simulink model "BBBC_5"  (R2022b)
settings: Solver=VariableStepAuto  StartTime=0.0  StopTime=5  RelTol=1e-3
undefined symbols (not defined in the file): dct, dEv, Ev, sigbuilder_block
libraries: simulink x6, spsMosfetLib x4, spsSeriesRLCBranchLib x4, spsCurrentMeasurementLib x2, spsVoltageMeasurementLib x2, spsGroundLib x1, spsControlledVoltageSourceLib x1, spspowerguiLib x1
settings Model: Creator=Dopechuro  LastModifiedBy=Dopechuro

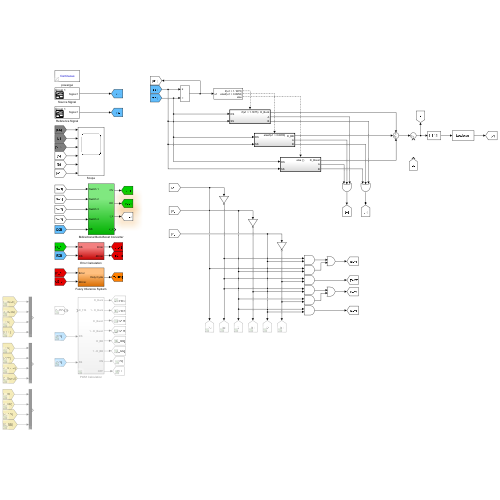
[thumbnail: Simulink's stored preview of the top-level diagram]
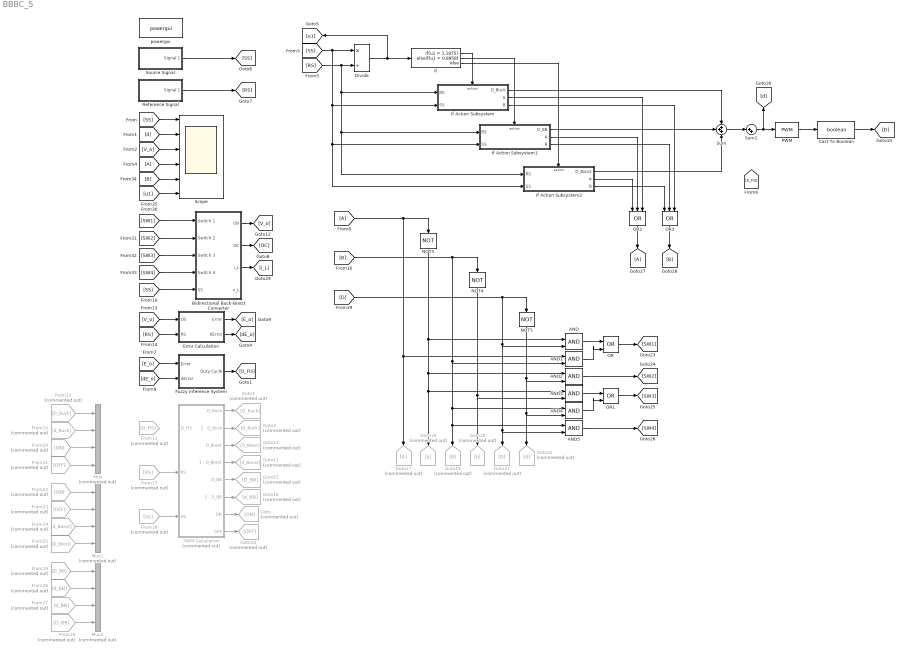
== system BBBC_5 ==
  AND{,1..5} (6 alike) : Logic  IconShape=distinctive  AllPortsSameDT=off  OutDataTypeStr=boolean
  Bidirectional Buck-Boost Converter : Subsystem
  Cast To Boolean : DataTypeConversion  OutDataTypeStr=boolean  SaturateOnIntegerOverflow=off  RndMeth=Floor
  Divide : Product  Inputs=*/
  Error Calculation : Subsystem
  From11 : From  Commented=on  GotoTag=D_FIS
  From12 : From  Commented=on  GotoTag=D_Buck
  From15 : From  Commented=on  GotoTag=d_Buck
  From17 : From  Commented=on  GotoTag=RS
  From18 : From  Commented=on  GotoTag=SS
  From19 : From  Commented=on  GotoTag=D_BB
  From20 : From  Commented=on  GotoTag=ON
  From21 : From  Commented=on  GotoTag=OFF
  From22 : From  Commented=on  GotoTag=ON
  From23 : From  Commented=on  GotoTag=OFF
  From24 : From  Commented=on  GotoTag=d_Boost
  From25 : From  Commented=on  GotoTag=D_Boost
  From26 : From  Commented=on  GotoTag=d_BB
  From27 : From  Commented=on  GotoTag=d_BB
  From28 : From  Commented=on  GotoTag=D_BB
  From4 : From
  From8 : From
  Fuzzy Inference System : Subsystem
  Goto : Goto  Commented=on  GotoTag=ON
  Goto11 : Goto  Commented=on  GotoTag=d_Boost
  Goto13 : Goto  Commented=on  GotoTag=D_Boost
  Goto14 : Goto  Commented=on  GotoTag=OFF
  Goto15 : Goto  Commented=on  GotoTag=D_BB
  Goto16 : Goto  Commented=on  GotoTag=d_BB
  Goto17 : Goto  Commented=on
  Goto18 : Goto  Commented=on  GotoTag=a
  Goto19 : Goto  Commented=on  GotoTag=B
  Goto2 : Goto  Commented=on  GotoTag=d_Buck
  Goto20 : Goto  Commented=on  GotoTag=b
  Goto21 : Goto  Commented=on  GotoTag=D
  Goto22 : Goto  Commented=on  GotoTag=d
  Goto27 : Goto
  Goto3 : Goto  Commented=on  GotoTag=D_Buck
  If : If  IfExpression=u1 > 1.1875  ElseIfExpressions=u1 > 0.8958
  If Action Subsystem : Subsystem  TreatAsAtomicUnit=on
  If Action Subsystem1 : Subsystem  TreatAsAtomicUnit=on
  If Action Subsystem2 : Subsystem  TreatAsAtomicUnit=on
  Mux : Mux  Commented=on
  Mux1 : Mux  Commented=on
  Mux2 : Mux  Commented=on
  NOT3 : Logic  Operator=NOT  IconShape=distinctive  AllPortsSameDT=off  OutDataTypeStr=boolean
  NOT4 : Logic  Operator=NOT  IconShape=distinctive  AllPortsSameDT=off  OutDataTypeStr=boolean
  NOT5 : Logic  Operator=NOT  IconShape=distinctive  AllPortsSameDT=off  OutDataTypeStr=boolean
  OR : Logic  Operator=OR  IconShape=distinctive  AllPortsSameDT=off  OutDataTypeStr=boolean
  OR1 : Logic  Operator=OR  IconShape=distinctive  AllPortsSameDT=off  OutDataTypeStr=boolean
  OR2 : Logic  Operator=OR  Inputs=3  IconShape=distinctive  AllPortsSameDT=off  OutDataTypeStr=boolean
  OR3 : Logic  Operator=OR  Inputs=3  IconShape=distinctive  AllPortsSameDT=off  OutDataTypeStr=boolean
  PWM : simulink/Discontinuities/PWM  DisableCoverage=on  Period=1e-5  InitialDelay=0  DisallowZeroDutyCycle=off  RunAtFixedTimeIntervals=off  SampleTime=0.1
  PWM Calculation : Subsystem  Commented=on
  Reference Signal : Subsystem  Tag=STV Subsys  LoadFcn=sigbuilder_block('load');  StartFcn=sigbuilder_block('start');  StopFcn=sigbuilder_block('stop');  ClipboardFcn=sigbuilder_block('clipboard');  mask(Sigbuilder block){tuvar=[0:10]}
      mask help: Simulink:masks:SigbuilderBlock_MD
      mask init:
      | if ~strcmp(get_param(bdroot(gcbh),'SimulationStatus'),'stopped') tuvar = sigbuilder_block('maskInit'); end
      settings: CopyFcn=sigbuilder_block('copy');  DeleteFcn=sigbuilder_block('delete');  ModelCloseFcn=sigbuilder_block('modelClose');  PreSaveFcn=sigbuilder_block('preSave');  PauseFcn=sigbuilder_block('pause');  ContinueFcn=sigbuilder_block('continue');  NameChangeFcn=sigbuilder_block('namechange');  OpenFcn=sigbuilder_block('open',[530.25 309.75 550.5 399.75 ]);  CloseFcn=sigbuilder_block('close');
      mask Display: plot(0, 0, 100, 100,[2, 2, 32, 32, 2], [68, 8, 8, 68, 68],[32, 2], [38, 38], [32, 19, 2],[53, 60, 44], [32, 17, 17, 2],[16, 16, 31, 31]);txt = getActiveGroup(gcbh);text(2, 100, txt,'verticalAlignment', 'top');
  Scope : Scope  NumInputPorts=6
  Source Signal : Subsystem  Tag=STV Subsys  LoadFcn=sigbuilder_block('load');  StartFcn=sigbuilder_block('start');  StopFcn=sigbuilder_block('stop');  ClipboardFcn=sigbuilder_block('clipboard');  mask(Sigbuilder block){tuvar=[0:10]}
      mask help: Simulink:masks:SigbuilderBlock_MD
      mask init:
      | if ~strcmp(get_param(bdroot(gcbh),'SimulationStatus'),'stopped') tuvar = sigbuilder_block('maskInit'); end
      settings: CopyFcn=sigbuilder_block('copy');  DeleteFcn=sigbuilder_block('delete');  ModelCloseFcn=sigbuilder_block('modelClose');  PreSaveFcn=sigbuilder_block('preSave');  PauseFcn=sigbuilder_block('pause');  ContinueFcn=sigbuilder_block('continue');  NameChangeFcn=sigbuilder_block('namechange');  OpenFcn=sigbuilder_block('open',[325.5 242.25 550.5 399.75 ]);  CloseFcn=sigbuilder_block('close');
      mask Display: plot(0, 0, 100, 100,[2, 2, 32, 32, 2], [68, 8, 8, 68, 68],[32, 2], [38, 38], [32, 19, 2],[53, 60, 44], [32, 17, 17, 2],[16, 16, 31, 31]);txt = getActiveGroup(gcbh);text(2, 100, txt,'verticalAlignment', 'top');
  Sum : Sum  Inputs=+++
  Sum1 : Sum  Inputs=|++
  powergui : spspowerguiLib/powergui  Priority=1  SimulationMode=Continuous  SampleTime=50e-6  frequency=60  Iterations=50  frequencyindice=0  Pbase=100e6  ErrMax=1e-4  UnitsV=kV  UnitsW=MW  buscounter=0  FunctionMessages=off  echomessages=off  EnableUseOfTLC=off  CurrentSourceSwitches=off  DisableSnubberDevices=off  DisableRonSwitches=off  DisableVfSwitches=off  DisplayEquations=off  AutomaticDiscreteSolvers=off  SolverType=Tustin/Backward Euler (TBE)  Interpol=off  ExternalGateDelay=off  methode=off  Ts=100  x0status=blocks  SPID=on  SwTol=0  HookPort=off  NonlinearTolerance=1e-4  nMaxIteration=100  ContinueOnMaxIteration=off  RestoreLinks=warning  ResistiveCurrentMeasurement=off  Frange=[0:2:500]  Ylog=off  Xlog=on  ShowGrid=off  save=off  variable=ZData  structure=0  ZoomFFT=off  StartTime=0.0  cycles=1  DisplayStyle=1  fundamental=60  FreqAxis=off  MaxFrequency=1000  frequencyindicesteady=1  RmsSteady=1  display=off
  wires:
  [d] -> Scope/2
  [V_o] -> Scope/3
  [V_o] -> Error Calculation/1(OS)
  [RS] -> Error Calculation/2(RS)
  Error Calculation/1(Error) -> [E_o]
  Error Calculation/2(dError) -> [dE_o]
  [SS] -> Scope/1
  [SS] -> Bidirectional Buck-Boost Converter/5(SS)
  Bidirectional Buck-Boost Converter/1(OV) -> [V_o]
  [E_o] -> Fuzzy Inference System/1(Error)
  [dE_o] -> Fuzzy Inference System/2(dError)
  Fuzzy Inference System/1(Duty Cycle) -> [D_FIS]
  [RS] -> If Action Subsystem/1(RS), If Action Subsystem2/1(RS), If Action Subsystem1/1(RS), Divide/2
  [SS] -> If Action Subsystem/2(SS), If Action Subsystem2/2(SS), If Action Subsystem1/2(SS), Divide/1
  From12/1 -> Mux/1
  From15/1 -> Mux/2
  From20/1 -> Mux/3
  From21/1 -> Mux/4
  From22/1 -> Mux1/1
  From23/1 -> Mux1/2
  From24/1 -> Mux1/3
  From25/1 -> Mux1/4
  From17/1 -> PWM Calculation/2(RS)
  From18/1 -> PWM Calculation/3(SS)
  PWM Calculation/2(1 - D_Buck) -> Goto2/1
  PWM Calculation/1(D_Buck) -> Goto3/1
  PWM Calculation/4(1 - D_Boost) -> Goto11/1
  PWM Calculation/7(ON) -> Goto/1
  PWM Calculation/8(OFF) -> Goto14/1
  PWM Calculation/3(D_Boost) -> Goto13/1
  PWM Calculation/5(D_BB) -> Goto15/1
  PWM Calculation/6(1 - D_BB) -> Goto16/1
  From28/1 -> Mux2/4
  From19/1 -> Mux2/1
  From27/1 -> Mux2/3
  From26/1 -> Mux2/2
  Bidirectional Buck-Boost Converter/2(OC) -> [OC]
  From4/1 -> Scope/4
  Divide/1 -> If/1, [u1]
  If/1 -> If Action Subsystem/Action
  If/2 -> If Action Subsystem1/Action
  If/3 -> If Action Subsystem2/Action
  If Action Subsystem1/1(D_BB) -> Sum/2
  If Action Subsystem/1(D_Buck) -> Sum/1
  If Action Subsystem2/1(D_Boost) -> Sum/3
  Sum/1 -> Sum1/1
  PWM/1 -> Cast To Boolean/1
  AND3/1 -> OR1/1
  [D] -> NOT5/1, AND5/2, Goto21/1, AND/2
  From8/1 -> AND1/1, Goto17/1, NOT3/1
  OR1/1 -> [SW3]
  AND1/1 -> OR/2
  AND4/1 -> OR1/2
  NOT4/1 -> Goto20/1, AND3/2
  [B] -> AND1/2, AND4/1, AND5/1, Goto19/1, NOT4/1
  AND5/1 -> [SW4]
  NOT5/1 -> Goto22/1, AND4/2, AND2/2
  OR/1 -> [SW1]
  NOT3/1 -> AND/1, AND2/1, AND3/1, Goto18/1
  AND2/1 -> [SW2]
  AND/1 -> OR/1
  If Action Subsystem/2(A) -> OR2/3
  If Action Subsystem1/2(A) -> OR2/2
  If Action Subsystem2/2(A) -> OR2/1
  If Action Subsystem/3(B) -> OR3/3
  If Action Subsystem1/3(B) -> OR3/2
  If Action Subsystem2/3(B) -> OR3/1
  OR2/1 -> Goto27/1
  Cast To Boolean/1 -> [D]
  Sum1/1 -> PWM/1, [d]
  [SW1] -> Bidirectional Buck-Boost Converter/1(Switch 1)
  [SW2] -> Bidirectional Buck-Boost Converter/2(Switch 2)
  [SW3] -> Bidirectional Buck-Boost Converter/3(Switch 3)
  [SW4] -> Bidirectional Buck-Boost Converter/4(Switch 4)
  Source Signal/1(Signal 1) -> [SS]
  Reference Signal/1(Signal 1) -> [RS]
  Bidirectional Buck-Boost Converter/3(i_L) -> [i_L]
  [B] -> Scope/5
  [u1] -> Scope/6
  OR3/1 -> [B]

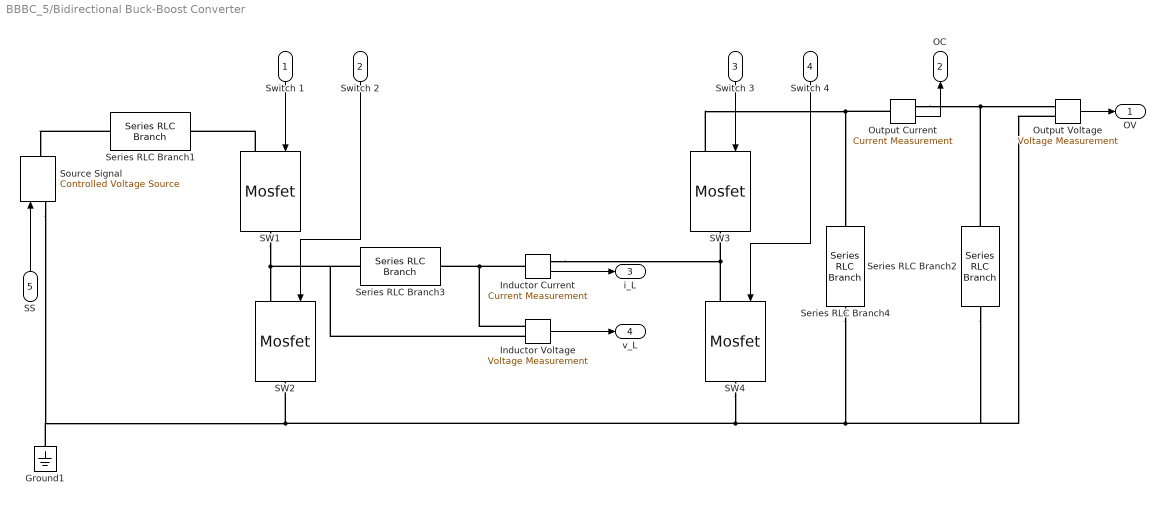
== system BBBC_5/Bidirectional Buck-Boost Converter ==
  Switch 1 : Inport
  Switch 2 : Inport  Port=2
  Switch 3 : Inport  Port=3
  Switch 4 : Inport  Port=4
  SS : Inport  Port=5
  Ground1 : spsGroundLib/Ground  LConnTagsString=a
  Inductor Current : spsCurrentMeasurementLib/Current Measurement  PhasorSimulation=off  OutputType=Complex  PSBequivalent=0
  Inductor Voltage : spsVoltageMeasurementLib/Voltage Measurement  PhasorSimulation=off  OutputType=Complex  PSBequivalent=0
  Output Current : spsCurrentMeasurementLib/Current Measurement  PhasorSimulation=off  OutputType=Complex  PSBequivalent=0
  Output Voltage : spsVoltageMeasurementLib/Voltage Measurement  PhasorSimulation=off  OutputType=Complex  PSBequivalent=0
  SW{1..4} (4 alike) : spsMosfetLib/Mosfet  Ron=0.1  Lon=0  Rd=0.01  Vfd=0  IC=0  Rs=1e5  Cs=inf  Measurements=off
  Series RLC Branch1 : spsSeriesRLCBranchLib/Series RLC Branch  LConnTagsString=__new0  RConnTagsString=__new0  BranchType=R  Resistance=0.1  Inductance=1e-3  SetiL0=off  InitialCurrent=0  Capacitance=1e-6  Setx0=off  InitialVoltage=0  Measurements=None
  Series RLC Branch2 : spsSeriesRLCBranchLib/Series RLC Branch  LConnTagsString=__new0  RConnTagsString=__new0  BranchType=R  Resistance=24  Inductance=1e-3  SetiL0=off  InitialCurrent=0  Capacitance=1000e-6  Setx0=off  InitialVoltage=0  Measurements=None
  Series RLC Branch3 : spsSeriesRLCBranchLib/Series RLC Branch  LConnTagsString=__new0  RConnTagsString=__new0  BranchType=RL  Resistance=0.1  Inductance=0.434e-3  SetiL0=off  InitialCurrent=0  Capacitance=1e-6  Setx0=off  InitialVoltage=0  Measurements=None
  Series RLC Branch4 : spsSeriesRLCBranchLib/Series RLC Branch  LConnTagsString=__new0  RConnTagsString=__new0  BranchType=RC  Resistance=0.01  Inductance=1e-3  SetiL0=off  InitialCurrent=0  Capacitance=10.6e-6  Setx0=off  InitialVoltage=0  Measurements=None
  Source Signal : spsControlledVoltageSourceLib/Controlled Voltage Source  Initialize=off  Source_Type=DC  Amplitude=0  Phase=0  Frequency=0  Measurements=None
  OV : Outport
  OC : Outport  Port=2
  i_L : Outport  Port=3
  v_L : Outport  Port=4
  wires:
  Switch 1/1 -> SW1/1
  Switch 3/1 -> SW3/1
  Switch 2/1 -> SW2/1
  SS/1 -> Source Signal/1
  Switch 4/1 -> SW4/1
  Inductor Current/1 -> i_L/1
  Output Voltage/1 -> OV/1
  Inductor Voltage/1 -> v_L/1
  Output Current/1 -> OC/1
  connections:
  SW1/LConn1 -- Series RLC Branch1/RConn1
  Inductor Current/LConn1 -- Inductor Voltage/LConn2 -- Series RLC Branch3/RConn1
  SW4/LConn1 -- Inductor Current/RConn1 -- SW3/RConn1
  SW4/RConn1 -- Output Voltage/LConn2 -- Series RLC Branch2/RConn1 -- Series RLC Branch4/RConn1 -- Source Signal/LConn1 -- Ground1/LConn1 -- SW2/RConn1
  SW1/RConn1 -- Inductor Voltage/LConn1 -- Series RLC Branch3/LConn1 -- SW2/LConn1
  Series RLC Branch1/LConn1 -- Source Signal/RConn1
  Output Current/RConn1 -- Output Voltage/LConn1 -- Series RLC Branch2/LConn1
  SW3/LConn1 -- Output Current/LConn1 -- Series RLC Branch4/LConn1

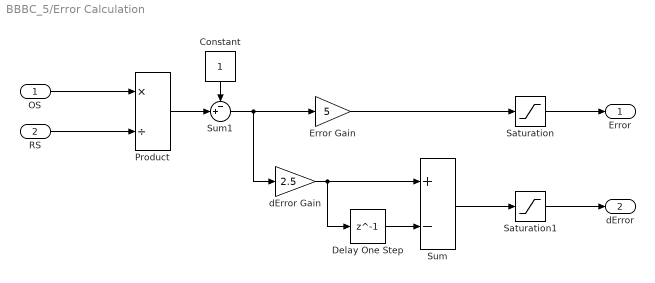
== system BBBC_5/Error Calculation ==
  OS : Inport
  RS : Inport  Port=2
  Constant : Constant
  Delay One Step : Delay  DelayLength=1
  Error Gain : Gain  Gain=5
  Product : Product  Inputs=*/
  Saturation : Saturate  UpperLimit=1  LowerLimit=-1
  Saturation1 : Saturate  UpperLimit=1  LowerLimit=-1
  Sum : Sum  Inputs=+-
  Sum1 : Sum  Inputs=-+|
  dError Gain : Gain  Gain=2.5
  Error : Outport
  dError : Outport  Port=2
  wires:
  Sum1/1 -> dError Gain/1, Error Gain/1
  dError Gain/1 -> Sum/1, Delay One Step/1
  Error Gain/1 -> Saturation/1
  Constant/1 -> Sum1/1
  Delay One Step/1 -> Sum/2
  Product/1 -> Sum1/2
  Sum/1 -> Saturation1/1
  OS/1 -> Product/1
  RS/1 -> Product/2
  Saturation/1 -> Error/1
  Saturation1/1 -> dError/1

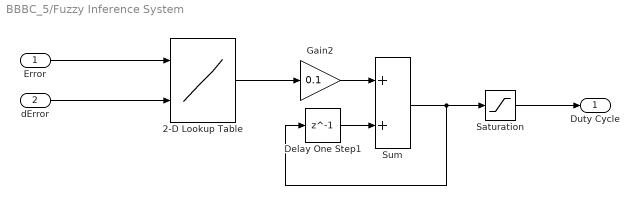
== system BBBC_5/Fuzzy Inference System ==
  Error : Inport
  dError : Inport  Port=2
  2-D Lookup Table : Lookup_n-D  LookupTableObject=''  BreakpointsForDimension1=Ev  BreakpointsForDimension2=dEv  BreakpointsForDimension1FirstPoint=10  BreakpointsForDimension2FirstPoint=10  BreakpointsForDimension1Spacing=12  BreakpointsForDimension2Spacing=12  IndexSearchMethod=Evenly spaced points  Table=dct  InterpMethod=Nearest  DiagnosticForOutOfRangeInput=Warning  InternalRulePriority=Speed  OutDataTypeStr=Inherit: Inherit from 'Table data'  RndMeth=Simplest
      settings: InputPortMap=u0,u1
  Delay One Step1 : Delay  DelayLength=1
  Gain2 : Gain  Gain=0.1
  Saturation : Saturate  UpperLimit=0.9  LowerLimit=-0.9
  Sum : Sum
  Duty Cycle : Outport
  wires:
  Delay One Step1/1 -> Sum/2
  Sum/1 -> Saturation/1, Delay One Step1/1
  Gain2/1 -> Sum/1
  2-D Lookup Table/1 -> Gain2/1
  Saturation/1 -> Duty Cycle/1
  Error/1 -> 2-D Lookup Table/1
  dError/1 -> 2-D Lookup Table/2

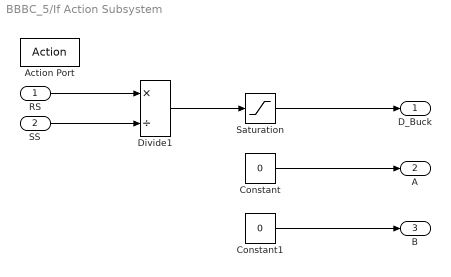
== system BBBC_5/If Action Subsystem ==
  RS : Inport
  SS : Inport  Port=2
  Action Port : ActionPort  ActionPortLabel=if(u1 > 1.1875)
  Constant : Constant  Value=0
  Constant1 : Constant  Value=0
  Divide1 : Product  Inputs=*/
  Saturation : Saturate  UpperLimit=0.85  LowerLimit=0.1
  D_Buck : Outport
  A : Outport  Port=2
  B : Outport  Port=3
  wires:
  Saturation/1 -> D_Buck/1
  RS/1 -> Divide1/1
  SS/1 -> Divide1/2
  Divide1/1 -> Saturation/1
  Constant1/1 -> B/1
  Constant/1 -> A/1

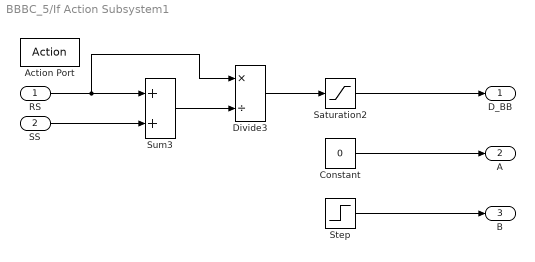
== system BBBC_5/If Action Subsystem1 ==
  RS : Inport
  SS : Inport  Port=2
  Action Port : ActionPort  ActionPortLabel=elseif(u1 > 0.8958)
  Constant : Constant  Value=0
  Divide3 : Product  Inputs=*/
  Saturation2 : Saturate  UpperLimit=0.85  LowerLimit=0.1
  Step : Step  Time=1e-9  SampleTime=0
  Sum3 : Sum
  D_BB : Outport
  A : Outport  Port=2
  B : Outport  Port=3
  wires:
  Saturation2/1 -> D_BB/1
  Sum3/1 -> Divide3/2
  RS/1 -> Sum3/1, Divide3/1
  SS/1 -> Sum3/2
  Divide3/1 -> Saturation2/1
  Step/1 -> B/1
  Constant/1 -> A/1

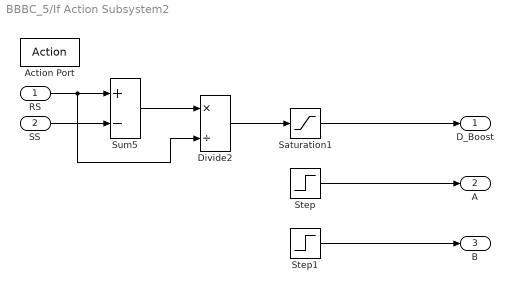
== system BBBC_5/If Action Subsystem2 ==
  RS : Inport
  SS : Inport  Port=2
  Action Port : ActionPort  ActionPortLabel=else
  Divide2 : Product  Inputs=*/
  Saturation1 : Saturate  UpperLimit=0.85  LowerLimit=0.1
  Step : Step  Time=1e-9  SampleTime=0
  Step1 : Step  Time=1e-9  SampleTime=0
  Sum5 : Sum  Inputs=+-
  D_Boost : Outport
  A : Outport  Port=2
  B : Outport  Port=3
  wires:
  Sum5/1 -> Divide2/1
  Divide2/1 -> Saturation1/1
  Saturation1/1 -> D_Boost/1
  RS/1 -> Divide2/2, Sum5/1
  SS/1 -> Sum5/2
  Step1/1 -> B/1
  Step/1 -> A/1

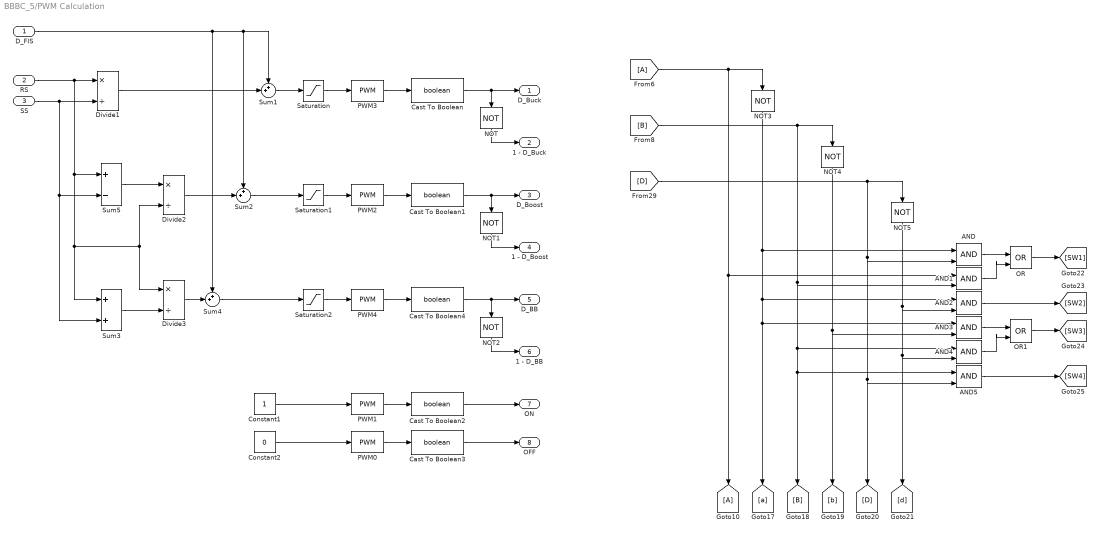
== system BBBC_5/PWM Calculation ==
  D_FIS : Inport
  RS : Inport  Port=2
  SS : Inport  Port=3
  AND{,1..5} (6 alike) : Logic  IconShape=distinctive  AllPortsSameDT=off  OutDataTypeStr=boolean
  Cast To Boolean{,1..4} (5 alike) : DataTypeConversion  OutDataTypeStr=boolean  SaturateOnIntegerOverflow=off  RndMeth=Floor
  Constant1 : Constant
  Constant2 : Constant  Value=0
  Divide1 : Product  Inputs=*/
  Divide2 : Product  Inputs=*/
  Divide3 : Product  Inputs=*/
  From6 : From
  Goto10 : Goto
  NOT{,1..5} (6 alike) : Logic  Operator=NOT  IconShape=distinctive  AllPortsSameDT=off  OutDataTypeStr=boolean
  OR : Logic  Operator=OR  IconShape=distinctive  AllPortsSameDT=off  OutDataTypeStr=boolean
  OR1 : Logic  Operator=OR  IconShape=distinctive  AllPortsSameDT=off  OutDataTypeStr=boolean
  PWM{0..4} (5 alike) : simulink/Discontinuities/PWM  DisableCoverage=on  Period=1/1e4  InitialDelay=0  DisallowZeroDutyCycle=off  RunAtFixedTimeIntervals=off  SampleTime=0.1
  Saturation : Saturate  UpperLimit=0.85  LowerLimit=0.1
  Saturation1 : Saturate  UpperLimit=0.85  LowerLimit=0.1
  Saturation2 : Saturate  UpperLimit=0.85  LowerLimit=0.1
  Sum1 : Sum  Inputs=++|
  Sum2 : Sum  Inputs=++|
  Sum3 : Sum
  Sum4 : Sum  Inputs=++|
  Sum5 : Sum  Inputs=+-
  D_Buck : Outport
  1 - D_Buck : Outport  Port=2
  D_Boost : Outport  Port=3
  1 - D_Boost : Outport  Port=4
  D_BB : Outport  Port=5
  1 - D_BB : Outport  Port=6
  ON : Outport  Port=7
  OFF : Outport  Port=8
  wires:
  Divide1/1 -> Sum1/2
  RS/1 -> Divide1/1, Sum5/1, Divide2/2, Divide3/1, Sum3/1
  SS/1 -> Divide1/2, Sum5/2, Sum3/2
  NOT/1 -> 1 - D_Buck/1
  Sum2/1 -> Saturation1/1
  PWM2/1 -> Cast To Boolean1/1
  NOT1/1 -> 1 - D_Boost/1
  PWM0/1 -> Cast To Boolean3/1
  PWM1/1 -> Cast To Boolean2/1
  PWM3/1 -> Cast To Boolean/1
  Sum1/1 -> Saturation/1
  Constant2/1 -> PWM0/1
  Constant1/1 -> PWM1/1
  D_FIS/1 -> Sum1/1, Sum2/1, Sum4/1
  Cast To Boolean/1 -> NOT/1, D_Buck/1
  Cast To Boolean1/1 -> NOT1/1, D_Boost/1
  Cast To Boolean2/1 -> ON/1
  Cast To Boolean3/1 -> OFF/1
  Saturation/1 -> PWM3/1
  Saturation1/1 -> PWM2/1
  Saturation2/1 -> PWM4/1
  PWM4/1 -> Cast To Boolean4/1
  Cast To Boolean4/1 -> NOT2/1, D_BB/1
  NOT2/1 -> 1 - D_BB/1
  Sum3/1 -> Divide3/2
  Divide3/1 -> Sum4/2
  Sum4/1 -> Saturation2/1
  Divide2/1 -> Sum2/2
  Sum5/1 -> Divide2/1
  AND2/1 -> [SW2]
  AND/1 -> OR/1
  NOT3/1 -> AND/1, AND2/1, AND3/1, [a]
  NOT5/1 -> [d], AND4/2, AND2/2
  [B] -> AND1/2, AND4/1, AND5/1, [B], NOT4/1
  AND1/1 -> OR/2
  AND5/1 -> [SW4]
  OR1/1 -> [SW3]
  From6/1 -> AND1/1, Goto10/1, NOT3/1
  [D] -> NOT5/1, AND5/2, [D], AND/2
  NOT4/1 -> [b], AND3/2
  AND3/1 -> OR1/1
  OR/1 -> [SW1]
  AND4/1 -> OR1/2

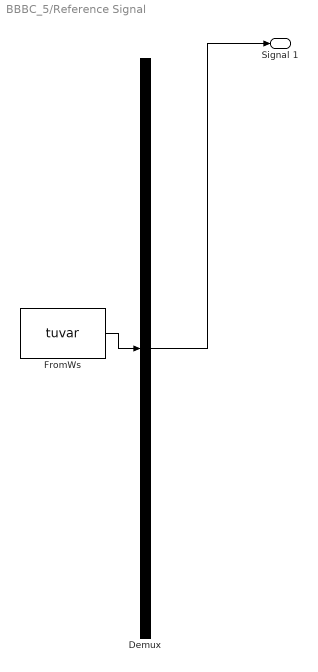
== system BBBC_5/Reference Signal ==
  Demux : Demux  Tag=STV Demux  Outputs=1
      settings: DisplayOption=none
  FromWs : FromWorkspace  Tag=STV FromWs  VariableName=tuvar
      SigBuilderData=|
      | common.afterFinalStr = 'Extrapolate'
      | common.sampleTime = 0
      | dataSet.timeRange = [0 5]
      | dataSet.name = 'Group 1'
      | sbobj.Groups.Name = 'Group 1'
      | sbobj.Groups.Signals.Name = 'Signal 1'
      | sbobj.Groups.Signals.XData = [0 5]
      | sbobj.Groups.Signals.YData = [48 48]
      | sbobj.Groups.TimeRange = [0 5]
  Signal 1 : Outport  Tag=STV Outport
  wires:
  FromWs/1 -> Demux/1
  Demux/1 -> Signal 1/1

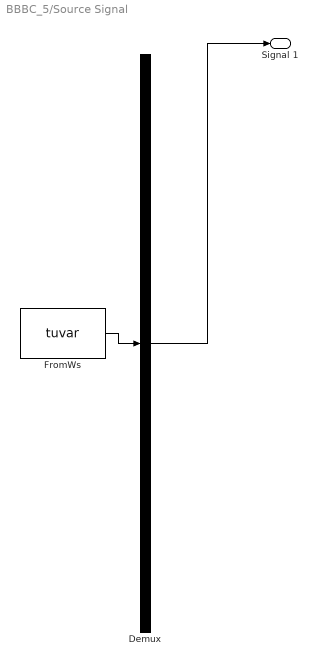
== system BBBC_5/Source Signal ==
  Demux : Demux  Tag=STV Demux  Outputs=1
      settings: DisplayOption=none
  FromWs : FromWorkspace  Tag=STV FromWs  VariableName=tuvar
      SigBuilderData=|
      | common.afterFinalStr = 'Extrapolate'
      | common.sampleTime = 0
      | dataSet.timeRange = [0 5]
      | dataSet.name = 'Group 1'
      | sbobj.Groups.Name = 'Group 1'
      | sbobj.Groups.Signals.Name = 'Signal 1'
      | sbobj.Groups.Signals.XData = [0 5]
      | sbobj.Groups.Signals.YData = [70 35]
      | sbobj.Groups.TimeRange = [0 5]
  Signal 1 : Outport  Tag=STV Outport
  wires:
  FromWs/1 -> Demux/1
  Demux/1 -> Signal 1/1
